simulink model "sim5"  (R2015b)
settings: Solver=VariableStepAuto  StartTime=0.0  StopTime=10.0  RelTol=1e-3
values from neighbouring files (symbols this model uses):
  beta = 0.001    [Lab3.m]    (also in calc_erro_l1.m; calc_erro_l2.m)
  dteta_inicial = 0    [Lab3.m]    (also in calc_erro_l1.m; calc_erro_l2.m)
  g = 9.8    [Lab3.m]    (also in calc_erro_l1.m; calc_erro_l2.m)
  J = (m*l^2)+(M/3)*L^2    (= 0.00626971061233)    [Lab3.m]    (also in fcn.m = (m*l^2)+(M/3)*L^2)
  k = 0.35    [Lab3.m]    (also in calc_erro_l1.m; calc_erro_l2.m; calc_media_BPM.m = 2)
  l = 0.2289    [Lab3.m]    (also in calc_erro_l1.m = x; calc_erro_l2.m = x; parametros_estimados.m = l_set(ind_c))
  L = 0.25    [Lab3.m]    (also in calc_erro_l1.m; calc_erro_l2.m)
  m = 0.0799    [Lab3.m]    (also in calc_erro_l1.m; calc_erro_l2.m; parametros_estimados.m = m_set(ind_r))
  M = 0.1    [Lab3.m]    (also in calc_erro_l1.m; calc_erro_l2.m)
  teta_inicial = pi/4    (= 0.785398163397)    [Lab3.m]    (also in calc_erro_l1.m; calc_erro_l2.m)
settings Model: Creator=Alice  LastModifiedBy=Alice

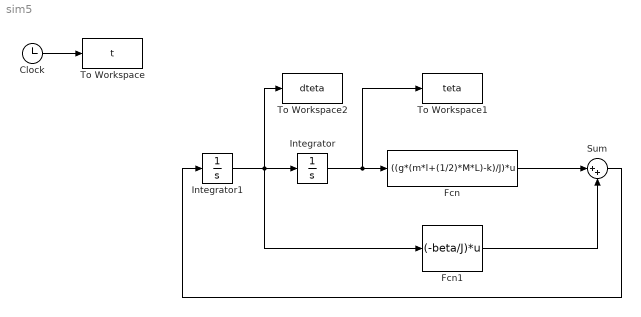
== system sim5 ==
  Clock : Clock
  Fcn : Fcn  Expr=((g*(m*l+(1/2)*M*L)-k)/J)*u
  Fcn1 : Fcn  Expr=(-beta/J)*u
  Integrator : Integrator  InitialCondition=teta_inicial
  Integrator1 : Integrator  InitialCondition=dteta_inicial
  Sum : Sum  Inputs=|++
  To Workspace : ToWorkspace  VariableName=t  SampleTime=0.01
  To Workspace1 : ToWorkspace  VariableName=teta  SampleTime=0.01
  To Workspace2 : ToWorkspace  VariableName=dteta  SampleTime=0.01
  wires:
  Integrator/1 -> To Workspace1/1, Fcn/1
  Integrator1/1 -> To Workspace2/1, Fcn1/1, Integrator/1
  Fcn/1 -> Sum/1
  Fcn1/1 -> Sum/2
  Sum/1 -> Integrator1/1
  Clock/1 -> To Workspace/1
